simulink model "Longitudinal_Autopilot_Jetstar_FC4_Testing_Linear_Model"  (R2020a)
settings: Solver=FixedStepAuto  StartTime=0.0  StopTime=300  FixedStep=0.01  RelTol=1e-3
values from neighbouring files (symbols this model uses):
  A_Long = [Xu                     , Xw                      , -w_0                         , -g*cos(theta_0) ... (first row only)    [Longitudinal_Linearized_Matrices.m]
  B_Long = [Xdel_e                          , Xdel_t ... (first row only)    [Longitudinal_Linearized_Matrices.m]
  C_Long = eye(4)    [Longitudinal_Linearized_Matrices.m]
  D_Long = zeros(4,2)    [Longitudinal_Linearized_Matrices.m]
undefined symbols (not defined in the file or in its folder): theta_0, u_0, w_0, z_0
libraries: cstblocks x3
settings Model: Creator=mohan  LastModifiedBy=mohan

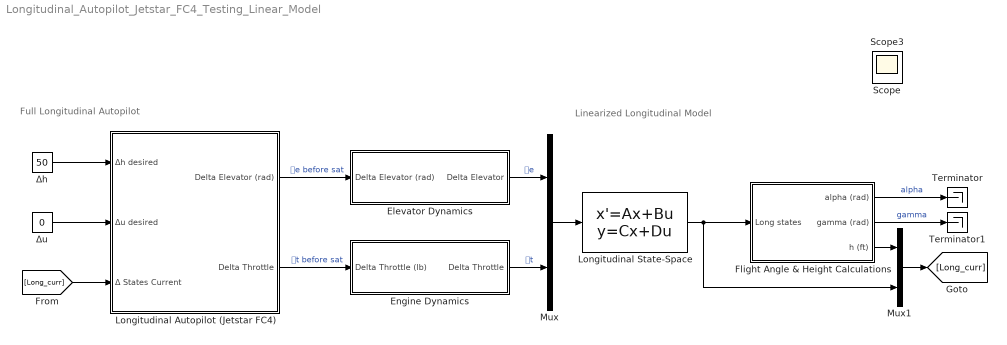
== system Longitudinal_Autopilot_Jetstar_FC4_Testing_Linear_Model ==
  note: Linearized Longitudinal Model
  note: Full Longitudinal Autopilot
  Elevator Dynamics : Subsystem  mask{delta_e_max=25}
      mask prompts: delta_e_max "Maximum Elevator Deflection (deg)"
      mask DialogControl ParameterGroupVar Prompt: Elevator Limits
  Engine Dynamics : Subsystem  mask{thrust_max=16000, thrust_min=-48000}
      mask prompts: thrust_max "Maximum Thrust"; thrust_min "Minimum Thrust"
      mask DialogControl ParameterGroupVar Prompt: Engine Limits
  Flight Angle & Height Calculations : Subsystem
  Longitudinal Autopilot (Jetstar FC4) : Subsystem  mask{Kp_alt=0.001862, Kd_alt=0.001694, Kp_pitch=1.6546, a_pitch=0.4868, Kd_pitch=0.52894, Kp_vel=1027.7, a_vel=0.05, Kd_vel=1523.9, zero_vel=0.1, pole_vel=0.7033}
      mask prompts: Kp_alt "Kp"; Kd_alt "Kd"; Kp_pitch "Kp"; a_pitch "a"; Kd_pitch "Kd"; Kp_vel "Kp"; a_vel "a"; Kd_vel "Kd"; zero_vel "Compensator Zero"; pole_vel "Compensator Pole"
      mask DialogControl ParameterGroupVar Prompt: Controllers
      mask DialogControl Container6 Prompt: Altitude Controller Gains (PD)
      mask DialogControl Container5 Prompt: Pitch Controller Gains (PID)
      mask DialogControl Container8 Prompt: Velocity Controller Gains (PI + Lead Compensator)
  Longitudinal State-Space : StateSpace  A=A_Long  B=B_Long  C=C_Long  D=D_Long  InitialCondition=[]
  Mux : Mux  Inputs=2
  Mux1 : Mux  Inputs=2
  Terminator : Terminator
  Terminator1 : Terminator
  Δh : Constant  Value=50
  Δu : Constant  Value=0
  Scope : Scope
  Scope3 : Scope
  wires:
  Mux/1 -> Longitudinal State-Space/1
  Longitudinal Autopilot (Jetstar FC4)/1(Delta Elevator (rad)) -> Elevator Dynamics/1(Delta Elevator (rad))  "𝛿e before sat"
  Longitudinal Autopilot (Jetstar FC4)/2(Delta Throttle) -> Engine Dynamics/1(Delta Throttle (lb))  "𝛿t before sat"
  Elevator Dynamics/1(Delta Elevator) -> Mux/1  "𝛿e"
  Engine Dynamics/1(Delta Throttle) -> Mux/2  "𝛿t"
  Longitudinal State-Space/1 -> Mux1/2, Flight Angle & Height Calculations/1(Long states)
  [Long_curr] -> Longitudinal Autopilot (Jetstar FC4)/3(Δ States Current)
  Δu/1 -> Longitudinal Autopilot (Jetstar FC4)/2(Δu desired)
  Δh/1 -> Longitudinal Autopilot (Jetstar FC4)/1(Δh desired)
  Mux1/1 -> [Long_curr]
  Flight Angle & Height Calculations/1(alpha (rad)) -> Terminator/1  "alpha"
  Flight Angle & Height Calculations/2(gamma (rad)) -> Terminator1/1  "gamma"
  Flight Angle & Height Calculations/3(h (ft)) -> Mux1/1

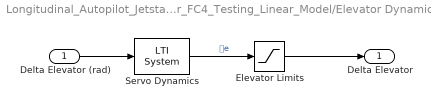
== system Longitudinal_Autopilot_Jetstar_FC4_Testing_Linear_Model/Elevator Dynamics ==
  Delta Elevator (rad) : Inport
  Elevator Limits : Saturate  UpperLimit=delta_e_max*pi/180  LowerLimit=-delta_e_max*pi/180
  Servo Dynamics : cstblocks/LTI System  sys=-tf(10,[1 10])  IC=[]
  Delta Elevator : Outport
  wires:
  Servo Dynamics/1 -> Elevator Limits/1  "𝛿e"
  Elevator Limits/1 -> Delta Elevator/1
  Delta Elevator (rad)/1 -> Servo Dynamics/1

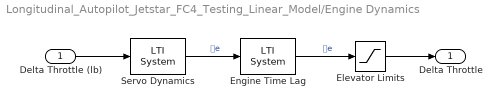
== system Longitudinal_Autopilot_Jetstar_FC4_Testing_Linear_Model/Engine Dynamics ==
  Delta Throttle (lb) : Inport
  Elevator Limits : Saturate  UpperLimit=thrust_max  LowerLimit=thrust_min
  Engine Time Lag : cstblocks/LTI System  sys=tf(0.1,[1 0.1])  IC=[]
  Servo Dynamics : cstblocks/LTI System  sys=tf(10,[1 10])  IC=[]
  Delta Throttle : Outport
  wires:
  Servo Dynamics/1 -> Engine Time Lag/1  "𝛿e"
  Elevator Limits/1 -> Delta Throttle/1
  Delta Throttle (lb)/1 -> Servo Dynamics/1
  Engine Time Lag/1 -> Elevator Limits/1  "𝛿e"

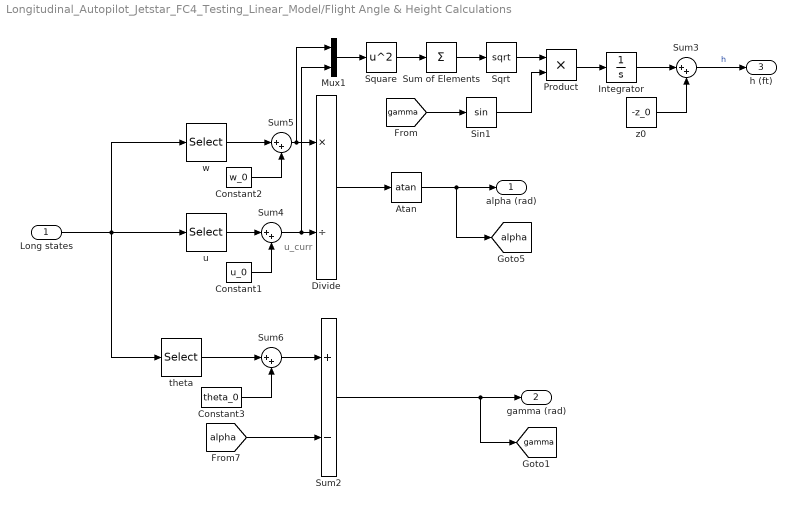
== system Longitudinal_Autopilot_Jetstar_FC4_Testing_Linear_Model/Flight Angle & Height Calculations ==
  note: u_curr
  Long states : Inport
  Atan : Trigonometry  Operator=atan
  Constant1 : Constant  Value=u_0
  Constant2 : Constant  Value=w_0
  Constant3 : Constant  Value=theta_0
  Divide : Product  Inputs=*/
  Integrator : Integrator
  Mux1 : Mux  Inputs=2
  Product : Product
  Sin1 : Trigonometry
  Sqrt : Sqrt  SaturateOnIntegerOverflow=on
  Square : Math  Operator=square  SaturateOnIntegerOverflow=on
  Sum of Elements : Sum  Inputs=+
  Sum2 : Sum  Inputs=+-
  Sum{3..6} (4 alike) : Sum  Inputs=|++
  theta : Selector  InputPortWidth=4  IndexOptions=Index vector (dialog)  Indices=4  OutputSizes=1
  u : Selector  InputPortWidth=4  IndexOptions=Index vector (dialog)  Indices=1  OutputSizes=1
  w : Selector  InputPortWidth=4  IndexOptions=Index vector (dialog)  Indices=2  OutputSizes=1
  z0 : Constant  Value=-z_0
  alpha (rad) : Outport
  gamma (rad) : Outport  Port=2
  h (ft) : Outport  Port=3
  tag scope: alpha=global, gamma=global
  wires:
  z0/1 -> Sum3/2
  Constant2/1 -> Sum5/2
  Sum2/1 -> [gamma], gamma (rad)/1
  u/1 -> Sum4/1
  [gamma] -> Sin1/1
  Constant1/1 -> Sum4/2
  Atan/1 -> alpha (rad)/1, [alpha]
  Mux1/1 -> Square/1
  Square/1 -> Sum of Elements/1
  Sqrt/1 -> Product/1
  Constant3/1 -> Sum6/2
  Long states/1 -> u/1, w/1, theta/1
  Sum4/1 -> Mux1/2, Divide/2
  Sum3/1 -> h (ft)/1  "h"
  Sum6/1 -> Sum2/1
  Sum5/1 -> Mux1/1, Divide/1
  Sum of Elements/1 -> Sqrt/1
  w/1 -> Sum5/1
  [alpha] -> Sum2/2
  Sin1/1 -> Product/2
  Divide/1 -> Atan/1
  theta/1 -> Sum6/1
  Product/1 -> Integrator/1
  Integrator/1 -> Sum3/1

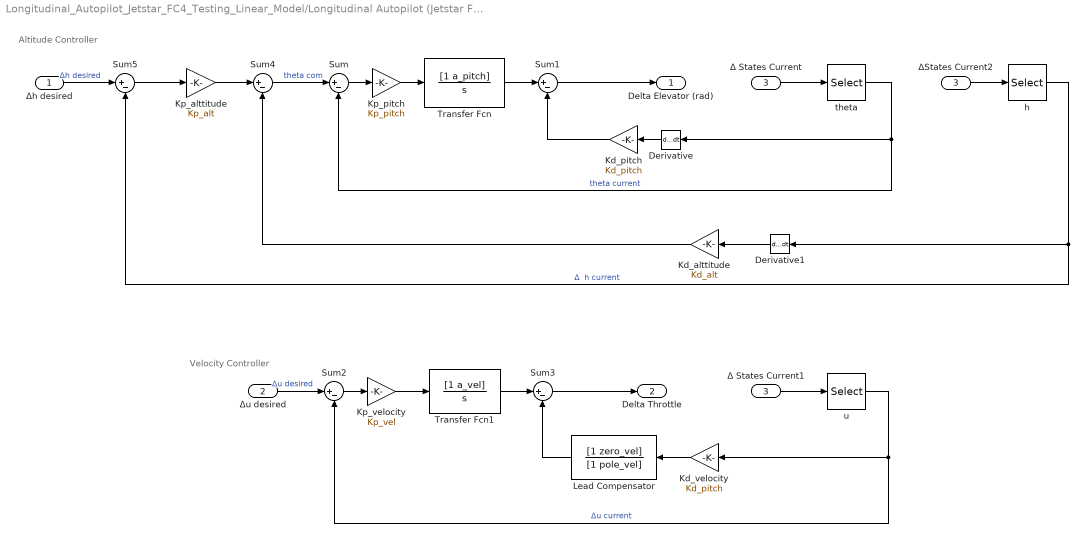
== system Longitudinal_Autopilot_Jetstar_FC4_Testing_Linear_Model/Longitudinal Autopilot (Jetstar FC4) ==
  note: Velocity Controller
  note: Altitude Controller
  Δh desired : Inport
  Δu desired : Inport  Port=2
  Δ States Current : Inport  Port=3
  Derivative : Derivative
  Derivative1 : Derivative
  Kd_alttitude : Gain  Gain=Kd_alt
  Kd_pitch : Gain  Gain=Kd_pitch
  Kd_velocity : Gain  Gain=Kd_pitch
  Kp_alttitude : Gain  Gain=Kp_alt
  Kp_pitch : Gain  Gain=Kp_pitch
  Kp_velocity : Gain  Gain=Kp_vel
  Lead Compensator : TransferFcn  Numerator=[1 zero_vel]  Denominator=[1 pole_vel]
  Sum{,1..5} (6 alike) : Sum  Inputs=|+-
  Transfer Fcn : TransferFcn  Numerator=[1 a_pitch]  Denominator=[1 0]
  Transfer Fcn1 : TransferFcn  Numerator=[1 a_vel]  Denominator=[1 0]
  h : Selector  InputPortWidth=5  IndexOptions=Index vector (dialog)  Indices=1  OutputSizes=1
  theta : Selector  InputPortWidth=5  IndexOptions=Index vector (dialog)  Indices=5  OutputSizes=1
  u : Selector  InputPortWidth=5  IndexOptions=Index vector (dialog)  Indices=2  OutputSizes=1
  Δ States Current1 : InportShadow  Port=3
  ΔStates Current2 : InportShadow  Port=3
  Delta Elevator (rad) : Outport
  Delta Throttle : Outport  Port=2
  wires:
  Transfer Fcn/1 -> Sum1/1
  Δ States Current/1 -> theta/1
  Sum4/1 -> Sum/1  "theta com"
  Kp_pitch/1 -> Transfer Fcn/1
  Sum/1 -> Kp_pitch/1
  Kd_pitch/1 -> Sum1/2
  Derivative/1 -> Kd_pitch/1
  Sum1/1 -> Delta Elevator (rad)/1
  Transfer Fcn1/1 -> Sum3/1
  Sum2/1 -> Kp_velocity/1
  Δ States Current1/1 -> u/1
  Kp_velocity/1 -> Transfer Fcn1/1
  Kd_velocity/1 -> Lead Compensator/1
  Δu desired/1 -> Sum2/1  "Δu desired"
  Sum3/1 -> Delta Throttle/1
  Lead Compensator/1 -> Sum3/2
  theta/1 -> Derivative/1, Sum/2  "theta current"
  u/1 -> Kd_velocity/1, Sum2/2  "Δu current"
  Sum5/1 -> Kp_alttitude/1
  Kd_alttitude/1 -> Sum4/2
  ΔStates Current2/1 -> h/1
  h/1 -> Derivative1/1, Sum5/2  "Δ  h current"
  Δh desired/1 -> Sum5/1  "Δh desired"
  Kp_alttitude/1 -> Sum4/1
  Derivative1/1 -> Kd_alttitude/1
